simulink model "Example_RPI_Xroad_exec"  (Simulink 3.00)
settings: Solver=ode45  SolverMode=SingleTasking  StartTime=0.0  StopTime=10.0  RelTol=1e-3
libraries: execlib x5
settings Model: ExtModeTrigMode=normal  ExtModeArmWhenConnect=on  Creator=ojezek  LastModifiedBy=XPMUser

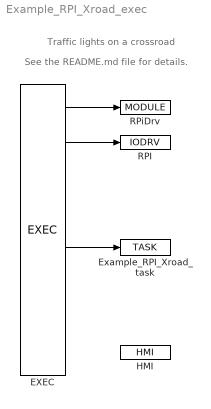
== system Example_RPI_Xroad_exec ==
  note: See the README.md file for details.
  note: Traffic lights on a crossroad
  EXEC : execlib/EXEC  target=Generic target device  tick=0.05  ntick0=2  ntick1=12  ntick2=15  ntick3=20  pri0=5  pri1=9  pri2=13  pri3=18
  Example_RPI_Xroad_task : execlib/TASK  factor=1  start=0  stop=1  stack=10240  MDLOPEN=on  bEdit=off
  HMI : execlib/HMI  IncludeHMI=on  HmiDir=hmi  SourceDir=hmisrc  GenerateWebWatch=on  GenerateRexHMI=on  RedirectToHMI=off  Compression=off  Compression=off  Compression=off  Compression=off  Compression=off  Compression=off
  RPI : execlib/IODRV  module=RPiDrv  classname=RPiDrv  factor=1  stack=10240  pri=3  timer=off
  RPiDrv : execlib/MODULE
  wires:
  EXEC/1 -> RPiDrv/1
  EXEC/2 -> RPI/1
  EXEC/5 -> Example_RPI_Xroad_task/1
